simulink model "ControllerStateModel_Harness1_replacement_Owner"  (R2024b)
settings: Solver=FixedStepAuto  StartTime=0.0  StopTime=10.0  FixedStep=0.01  RelTol=1e-3
undefined symbols (not defined in the file or in its folder): ALT_THRESHOLD, CLIMB_PITCH_CMD, GAIN, PERSISTENCT, STALL_SPEED
libraries: simulink x2
settings Model: DataDictionary=ControllerModel.sldd  Creator=MBD_PRO  LastModifiedBy=MBD_PRO

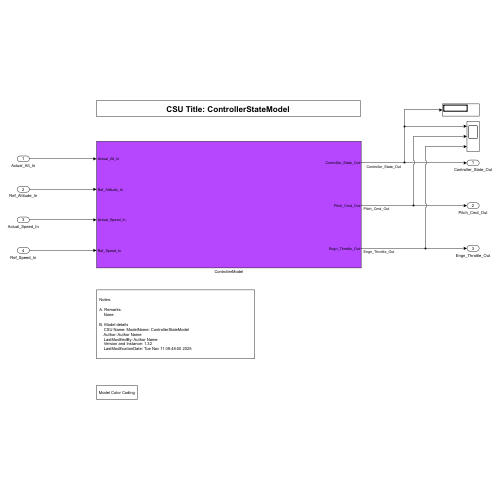
[thumbnail: Simulink's stored preview of the top-level diagram]
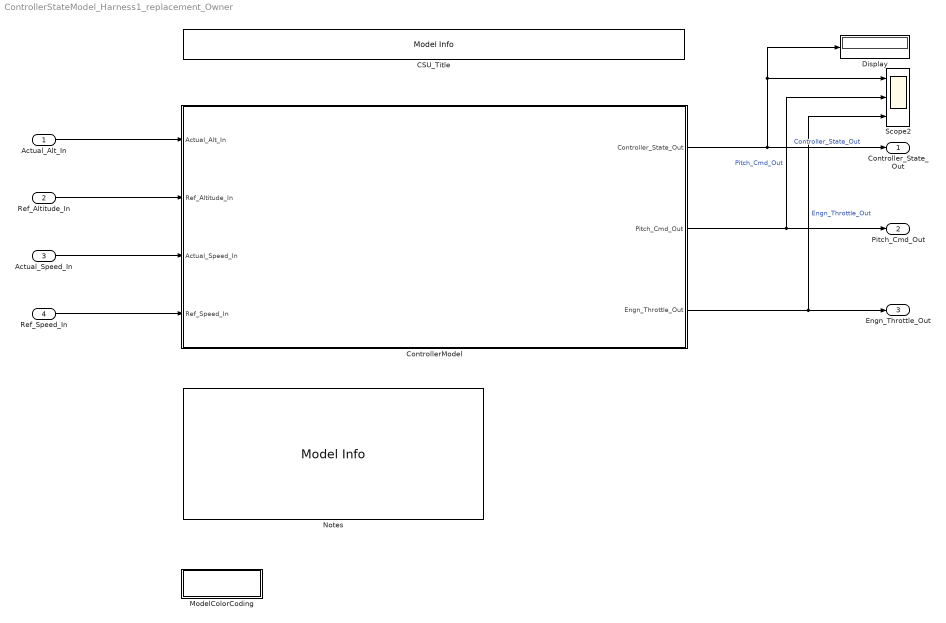
== system ControllerStateModel_Harness1_replacement_Owner ==
  Actual_Alt_In : Inport
  Ref_Altitude_In : Inport  Port=2
  Actual_Speed_In : Inport  Port=3
  Ref_Speed_In : Inport  Port=4
  CSU_Title : simulink/Model-Wide Utilities/Model Info  Frame=on  DisplayStringWithTags=CSU Title: %<ModelName>  HorizontalTextAlignment=Center  LeftAlignmentValue=0.5
  ControllerModel : Subsystem
  Display : Display
  ModelColorCoding : Subsystem
      mask Display: disp("Model Color Coding");
  Notes : simulink/Model-Wide Utilities/Model Info  Frame=on  DisplayStringWithTags=|  HorizontalTextAlignment=Left  LeftAlignmentValue=0.02
      | Notes:
      | 
      | A. Remarks:
      |     None
      | 
      | B. Model details
      |     CSU Name: ModelName: %<ModelName>
      |     Author: Author Name
      |     LastModifiedBy: Author Name
      |     Version and Instance: %<ModelVersion>
      |     LastModificationDate: %<LastModificationDate>
  Scope2 : Scope  NumInputPorts=3
  Controller_State_Out : Outport
  Pitch_Cmd_Out : Outport  Port=2
  Engn_Throttle_Out : Outport  Port=3
  wires:
  Actual_Speed_In/1 -> ControllerModel/3(Actual_Speed_In)
  Actual_Alt_In/1 -> ControllerModel/1(Actual_Alt_In)
  Ref_Speed_In/1 -> ControllerModel/4(Ref_Speed_In)
  Ref_Altitude_In/1 -> ControllerModel/2(Ref_Altitude_In)
  ControllerModel/1(Controller_State_Out) -> Display/1, Scope2/1, Controller_State_Out/1  "Controller_State_Out"
  ControllerModel/3(Engn_Throttle_Out) -> Scope2/3, Engn_Throttle_Out/1  "Engn_Throttle_Out"
  ControllerModel/2(Pitch_Cmd_Out) -> Scope2/2, Pitch_Cmd_Out/1  "Pitch_Cmd_Out"

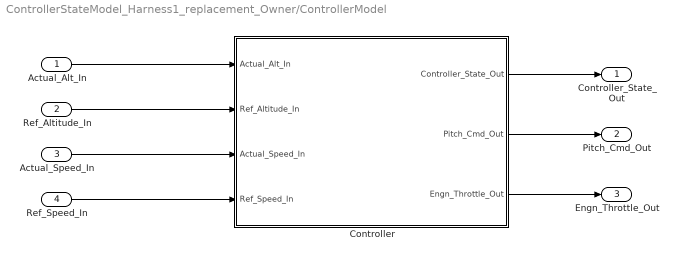
== system ControllerStateModel_Harness1_replacement_Owner/ControllerModel ==
  Actual_Alt_In : Inport
  Ref_Altitude_In : Inport  Port=2
  Actual_Speed_In : Inport  Port=3
  Ref_Speed_In : Inport  Port=4
  Controller : Stateflow chart  TreatAsAtomicUnit=on
  Controller_State_Out : Outport
  Pitch_Cmd_Out : Outport  Port=2
  Engn_Throttle_Out : Outport  Port=3
  wires:
  Controller/1(Controller_State_Out) -> Controller_State_Out/1
  Ref_Speed_In/1 -> Controller/4(Ref_Speed_In)
  Actual_Speed_In/1 -> Controller/3(Actual_Speed_In)
  Actual_Alt_In/1 -> Controller/1(Actual_Alt_In)
  Ref_Altitude_In/1 -> Controller/2(Ref_Altitude_In)
  Controller/2(Pitch_Cmd_Out) -> Pitch_Cmd_Out/1
  Controller/3(Engn_Throttle_Out) -> Engn_Throttle_Out/1

== system ControllerStateModel_Harness1_replacement_Owner/ModelColorCoding ==
  note: Model color coding
      |
      | Inport and Outport blocks color ( Cyan )
      | #00ffff
      |
      | Simulink Library blocks color (White)
      | #ffffff
      |
      | FCS ADE Library blocks color (Purple)
      | #00cc00
      |
      | Goto and From blocks color (Yellow)
      | #ffff00
      |
      | Disabled Link Library blocks color (Gray)
      | #ff7c7e
      |
      | Internal Subsystem color (Blue)
      | #55aaff
      |
      | Embeded matlab function (Gray)
      | #a6a6a6
      |
      | Outer Subsystem color (TBD)
      | #b746ff
      |
      | Model Reference block color (Orange)
      | #ff6929
      |
      | Any Remark or Note to the block color(TBD)
      | #aa0000

== stateflow chart ControllerStateModel_Harness1_replacement_Owner/ControllerModel/Controller ==
  state Normal
    entry:
    Controller_State_Out = Controller.Normal;
    count_stall_recov = 1;
    count_climb = 1;
    during:
    %
    % Transition from state Normal to Climb
    if ((Ref_Altitude_In - Actual_Alt_In) >= ALT_THRESHOLD)
    if (count_climb >= PERSISTENCT)
    Controller_State_Out = Controller.Climb;
    else
    count_climb = count_climb + 1;
    end
    else
    count_climb = 1;
    end
    %
    % Transition from state Normal to StallRecovery
    if Actual_Speed_In < STALL_SPEED
    if (count_stall_recov >= PERSISTENCT)
    Controller_State_Out = Controller.StallRecovery;
    else
    count_stall_recov = count_stall_recov + 1;
    end
    else
    count_stall_recov = 1;
    end
    %
    % Computation
    Pitch_Cmd_Out = (Ref_Altitude_In - Actual_Alt_In) * GAIN;
    Engn_Throttle_Out = (Ref_Speed_In - Actual_Speed_In) * GAIN;
    exit:
  state Climb
    entry:
    Controller_State_Out = Controller.Climb
    count_stall_recov = 1;
    count_normal = 1;
    during:
    %
    % Transition from state Climb to Normal
    if Actual_Alt_In > Ref_Altitude_In
    if (count_normal >= PERSISTENCT)
    Controller_State_Out = Controller.Normal;
    else
    count_normal = count_normal + 1;
    end
    else
    count_normal = 1;
    end
    %
    % Transition from state Climb to StallRecovery
    if Actual_Speed_In < STALL_SPEED
    if (count_stall_recov >= PERSISTENCT)
    Controller_State_Out = Controller.StallRecovery;
    else
    count_stall_recov = count_stall_recov + 1;
    end
    else
    count_stall_recov = 1;
    end
    %
    % Computation
    Pitch_Cmd_Out = CLIMB_PITCH_CMD;
    Engn_Throttle_Out = 100.0;
    exit:
  state StallRecovery
    entry:
    Controller_State_Out = Controller.StallRecovery
    count_climb = 1;
    during:
    % Transition from state StallRecovery to Normal
    if Actual_Speed_In > STALL_SPEED
    if (count_climb >= PERSISTENCT)
    Controller_State_Out = Controller.Normal;
    else
    count_climb = count_climb + 1;
    end
    else
    count_climb = 1;
    end
    % Computation
    Pitch_Cmd_Out = 0.0;
    Engn_Throttle_Out = 100.0;
    exit:
  (default) -> Normal
  Climb -> Normal [order 2] : [Controller_State_Out == Controller.Normal]
  Normal -> Climb [order 2] : [Controller_State_Out == Controller.Climb]
  StallRecovery -> Normal : [Controller_State_Out == Controller.Normal]
  Normal -> StallRecovery [order 1] : [Controller_State_Out == Controller.StallRecovery]
  Climb -> StallRecovery [order 1] : [Controller_State_Out == Controller.StallRecovery]
  data: Actual_Alt_In input; Ref_Altitude_In input; Actual_Speed_In input; Ref_Speed_In input; PERSISTENCT parameter double; Controller_State_Out output; STALL_SPEED parameter; count_stall_recov local; count_climb local; count_normal local; Pitch_Cmd_Out output =0.0; Engn_Throttle_Out output =0.0; GAIN parameter; CLIMB_PITCH_CMD parameter; ALT_THRESHOLD parameter
